simulink model "lab1sim"  (R2025b)
settings: Solver=VariableStepAuto  StartTime=0.0  StopTime=10.0  RelTol=1e-3
InitFcn:
  | m=1;
  | g=9.81;
  | l=1.5;
  | B=1.96;
settings Model: Creator=janek  LastModifiedBy=janek

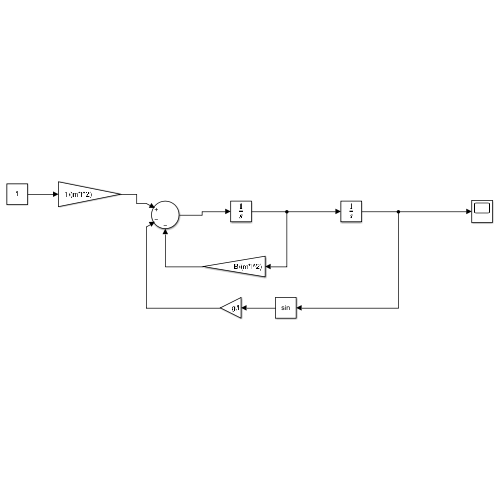
[thumbnail: Simulink's stored preview of the top-level diagram]
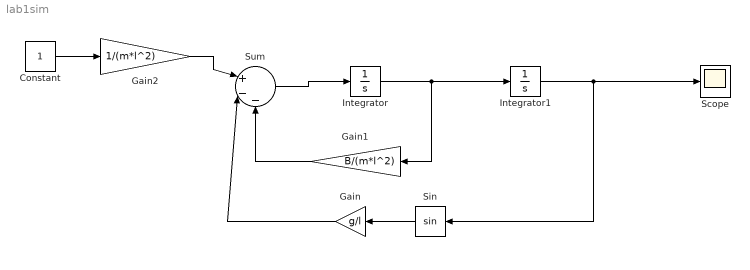
== system lab1sim ==
  Constant : Constant
  Gain : Gain  Gain=g/l
  Gain1 : Gain  Gain=B/(m*l^2)
  Gain2 : Gain  Gain=1/(m*l^2)
  Integrator : Integrator
  Integrator1 : Integrator
  Scope : Scope
  Sin : Trigonometry
  Sum : Sum  Inputs=|+--
  wires:
  Sum/1 -> Integrator/1
  Integrator/1 -> Gain1/1, Integrator1/1
  Integrator1/1 -> Sin/1, Scope/1
  Sin/1 -> Gain/1
  Gain/1 -> Sum/2
  Gain1/1 -> Sum/3
  Gain2/1 -> Sum/1
  Constant/1 -> Gain2/1
